simulink model "CartPole_env"  (R2023a)
settings: Solver=ode3  StartTime=0.0  StopTime=20.0  FixedStep=0.001  RelTol=1e-3  EnableMultiTasking=on
InitFcn:
  | Mp = 0.05;
  | Mc = 1;
  | l = 20; %half of the pole's length (distance from pivot to the center of mass of the pole)
  | g = 9.81;
libraries: simulink x1
settings Model: Creator=divij  LastModifiedBy=divij
settings DataIOCC: SaveFormat=Structure
settings OptimizationCC: ZeroExternalMemoryAtStartup=off  ZeroInternalMemoryAtStartup=off
settings RTWCC: PackageGeneratedCodeAndArtifacts=on  Toolchain=Catkin  BuildConfiguration=Debug  TargetLang=C++
settings GRTTargetCC: TargetLangStandard=C++11 (ISO)  MatFileLogging=off  CodeInterfacePackaging=C++ class

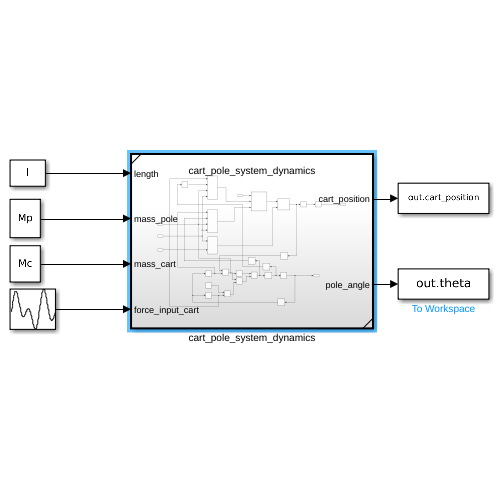
[thumbnail: Simulink's stored preview of the top-level diagram]
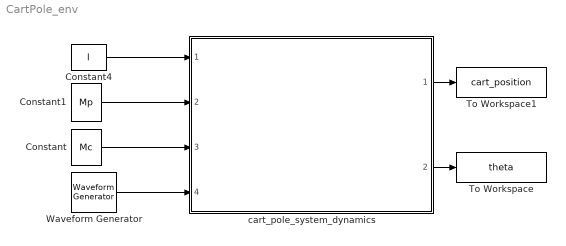
== system CartPole_env ==
  Constant : Constant  Value=Mc
  Constant1 : Constant  Value=Mp
  Constant4 : Constant  Value=l
  To Workspace : ToWorkspace  VariableName=theta  SaveFormat=Timeseries  SampleTime=-1
  To Workspace1 : ToWorkspace  VariableName=cart_position  SaveFormat=Timeseries  SampleTime=-1
  Waveform Generator : simulink/Sources/Waveform Generator  OutMin=[]  OutMax=[]  OutDataTypeStr=double  SelectedSignal=1  Signals=sin('Amplitude', 1, 'Frequency', 1, 'Phase', 1)  BlockNames=MultiportSwitch_5e66181ff19049d  SampleTime=0.1
  cart_pole_system_dynamics : Subsystem  TreatAsAtomicUnit=on  ReferencedSubsystem=cart_pole_system_dynamics
  wires:
  cart_pole_system_dynamics/1 -> To Workspace1/1
  cart_pole_system_dynamics/2 -> To Workspace/1
  Waveform Generator/1 -> cart_pole_system_dynamics/4
  Constant1/1 -> cart_pole_system_dynamics/2
  Constant4/1 -> cart_pole_system_dynamics/1
  Constant/1 -> cart_pole_system_dynamics/3
